simulink model "transmit_model"  (R2020a)
settings: Solver=VariableStepAuto  StartTime=0.0  StopTime=10.0  RelTol=1e-3
settings Model: Creator=24547  LastModifiedBy=24547

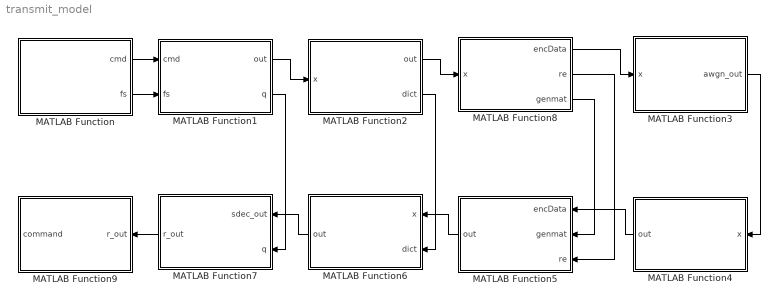
== system transmit_model ==
  MATLAB Function : MATLAB Function  TreatAsAtomicUnit=on
  MATLAB Function1 : MATLAB Function  TreatAsAtomicUnit=on
  MATLAB Function2 : MATLAB Function  TreatAsAtomicUnit=on
  MATLAB Function3 : MATLAB Function  TreatAsAtomicUnit=on
  MATLAB Function4 : MATLAB Function  TreatAsAtomicUnit=on
  MATLAB Function5 : MATLAB Function  TreatAsAtomicUnit=on
  MATLAB Function6 : MATLAB Function  TreatAsAtomicUnit=on
  MATLAB Function7 : MATLAB Function  TreatAsAtomicUnit=on
  MATLAB Function8 : MATLAB Function  TreatAsAtomicUnit=on
  MATLAB Function9 : MATLAB Function  TreatAsAtomicUnit=on
  wires:
  MATLAB Function/1(cmd) -> MATLAB Function1/1(cmd)
  MATLAB Function/2(fs) -> MATLAB Function1/2(fs)
  MATLAB Function1/1(out) -> MATLAB Function2/1(x)
  MATLAB Function2/1(out) -> MATLAB Function8/1(x)
  MATLAB Function8/1(encData) -> MATLAB Function3/1(x)
  MATLAB Function3/1(awgn_out) -> MATLAB Function4/1(x)
  MATLAB Function4/1(out) -> MATLAB Function5/1(encData)
  MATLAB Function8/3(genmat) -> MATLAB Function5/2(genmat)
  MATLAB Function8/2(re) -> MATLAB Function5/3(re)
  MATLAB Function5/1(out) -> MATLAB Function6/1(x)
  MATLAB Function2/2(dict) -> MATLAB Function6/2(dict)
  MATLAB Function6/1(out) -> MATLAB Function7/1(sdec_out)
  MATLAB Function1/2(q) -> MATLAB Function7/2(q)
  MATLAB Function7/1(r_out) -> MATLAB Function9/1(r_out)

== matlab function transmit_model/MATLAB Function1 ==
  data: out output; q output; cmd input; fs input
function [out, q] = quantize(cmd, fs)
%%% input
% N: 量化bit
% infile: 输入声音信号
%%% output
% out: 量化后的信号,0:2^N-1

N = 8
q = (1-(-1))/2^N;
out = floor((cmd+1)/q);

% 原始信号
len = length(cmd);
ts = (0:len-1)/fs;
figure;
plot(ts, cmd, 'r');
title('原始信号');
xlabel('time(s)');
ylabel('amplitude(V)');

% 重建信号
% reconstruct = q*out-1;
% figure;
% plot(ts, reconstruct, 'b')
% title('重建信号');
% xlabel('time(s)');
% cmdlabel('amplitude(V)');
end

== matlab function transmit_model/MATLAB Function ==
  data: cmd output; fs output
function [cmd, fs] = commandCreate
fs = 16000; 
R = audiorecorder(fs, 16 ,1) ;
disp('Start speaking.')
recordblocking(R,1);
disp('End of Recording.');
cmd = getaudiodata(R);
audiowrite('cmd.flac', cmd, fs);
end

== matlab function transmit_model/MATLAB Function2 ==
  data: out output; dict output; x input
function [out, dict] = source_encode(x)
%%% input
% x: 量化后的信号
% N: 量化bit
%%% output
% out: 哈夫曼编码结果

N = 8
len = length(x);
unique_x = unique(x);
unique_len = length(unique_x);

symbols = cell(1, unique_len);
p = zeros(1, unique_len);

% 计算符号概率
for i = 1:unique_len
    symbols{1,i} = unique_x(i);
    p(i) = numel(find(x==unique_x(i))) / len;
end

% 根据符号集symbols和概率数组p计算Huffman编码词典
[dict, avglen] = huffmandict(symbols, p);

fprintf('-------- source encode --------\n');

% 打印字典表
for i = 1:unique_len
    fprintf('%d : ', unique_x(i));
    fprintf('%d ', dict{i,2});
    fprintf('\n');
end

fprintf('平均码长 : %f\n', avglen );
fprintf('信源熵 : %f\n', sum(p.*(-log2(p))) );
fprintf('编码效率 : %f\n', 1/sum(p.*(-log2(p))) );

% 编码结果
out = huffmanenco(x, dict);

% 计算字符串最终编码长度
enc_len = length(out);

% 原始编码长度
len_before_enc = len*N;

fprintf('编码前字符串总长度 : %d\n', len_before_enc);
fprintf('编码后字符串二进制总长度 : %d\n', enc_len);
fprintf('压缩率 : %f\n', len_before_enc/enc_len);

% 打印最终编码
% fprintf('编码结果 : ');
% for i = 1:len
%     %fprintf('%s : ', x(i));
%     fprintf('%d', dict{unique_x==x(i),2});
%     fprintf(' ');
% end
% fprintf('\n');
end

== matlab function transmit_model/MATLAB Function3 ==
  data: awgn_out output; x input
function awgn_out  = modulation(x)
%%% QPSK modulation and AWGN
snr = 10;
qpsk_out = pskmod(x,4,pi/4);
awgn_out = awgn(qpsk_out, snr);
end

== matlab function transmit_model/MATLAB Function4 ==
  data: out output; x input
function out  = demodulation(x)
out = pskdemod(x,4,pi/4);
out = double(out > 0.5);
end

== matlab function transmit_model/MATLAB Function5 ==
  data: out output; encData input; genmat input; re input
function out  = channel_decode(encData, genmat, re)
n = 7;
k = 4;
encData = reshape(encData, n, length(encData)/n)';
decData = decode(encData,n,k,'linear/binary',genmat);
decData = reshape(decData', [], 1);
out = decData(1:(length(decData)-k+re));
end

== matlab function transmit_model/MATLAB Function6 ==
  data: out output; x input; dict input
function out  = source_decode(x, dict)
out = huffmandeco(x, dict);
end

== matlab function transmit_model/MATLAB Function7 ==
  data: r_out output; sdec_out input; q input
function r_out  = restore(sdec_out, q)
r_out = q*sdec_out-1;
figure;
plot(r_out, 'b')
title('重建信号');
xlabel('time(s)');
ylabel('amplitude(V)');
end

== matlab function transmit_model/MATLAB Function8 ==
  data: encData output; re output; x input; genmat output
function [encData, re, genmat] = channel_encode(x)
%%% input
% x: 信源编码后的结果
% n: 编码长度
% k: 信息长度
%%% output:
% encData: 线性分组码编码结果
% re: 余数
% genmat: 生成多项式

n = 7;
k = 4;
len = length(x);
data = zeros(ceil(len/k)*k, 1);
data(1:len) = x;
re = rem(len, k);
data = reshape(data, k, length(data)/k)';

pol = cyclpoly(n,k);
parmat = cyclgen(n,pol);
genmat = gen2par(parmat);
encData = encode(data,n,k,'linear/binary',genmat);
encData = reshape(encData', [], 1);

fprintf('-------- channel encode --------\n');
fprintf('生成多项式为: \n');
for i = 1:k
    fprintf('%d ', genmat(i, :));
    fprintf('\n');
end

end

== matlab function transmit_model/MATLAB Function9 ==
  data: command output; r_out input
function command = recognize(r_out)
load('commandNet.mat');
auditorySpect = helperExtractAuditoryFeatures(r_out,fs);
command = classify(trainedNet,auditorySpect);
disp(command)
end
